simulink model "clik_z_inverse"  (R2022b)
settings: Solver=ode1  StartTime=0.0  StopTime=4  FixedStep=0.001  RelTol=1e-3
undefined symbols (not defined in the file or in its folder): DiscIntNeverNeededParam, q0, Tc
settings Model: Creator=Xp  LastModifiedBy=reube
settings SolverCC: AlgebraicLoopSolver=TrustRegion
settings DataIOCC: LimitDataPoints=on  SaveFormat=Array  SignalLoggingSaveFormat=ModelDataLogs  ReturnWorkspaceOutputs=off
settings OptimizationCC: ExpressionDepthLimit=2147483647  InitFltsAndDblsToZero=on  LifeSpan=inf
settings DebuggingCC: SaveWithParameterizedLinksMsg=none  UnderspecifiedInitializationDetection=Classic  MergeDetectMultiDrivingBlocksExec=none  SolverPrmCheckMsg=warning  MultiTaskDSMMsg=warning  MultiTaskCondExecSysMsg=none  FcnCallInpInsideContextMsg=warning  UnconnectedInputMsg=warning  UnconnectedOutputMsg=warning  UnconnectedLineMsg=warning  StateNameClashWarn=warning  SFUnexpectedBacktrackingDiag=warning  SFNoUnconditionalDefaultTransitionDiag=warning  SFExecutionAtInitializationDiag=none  SFMachineParentedDataDiag=warning  ArithmeticOperatorsInVariantConditions=warning
settings HardwareCC: ProdBitPerPointer=32  ProdBitPerSizeT=32  ProdBitPerPtrDiffT=32  ProdLargestAtomicFloat=None  ProdIntDivRoundTo=Undefined  ProdEndianess=Unspecified  ProdWordSize=32  ProdHWDeviceType=32-bit Generic
settings ModelReferenceCC: EnableRefExpFcnMdlSchedulingChecks=on  PropagateSignalLabelsOutOfModel=off
settings SFSimCC: CustomCodeUndefinedFunction=UseInterfaceOnly
settings RTWCC: DLArmComputeVersion=19.05
settings CodeAppCC: StateflowObjectComments=on
settings GRTTargetCC: TargetLangStandard=C89/C90 (ANSI)  CombineOutputUpdateFcns=off  GRTInterface=on
settings ConfigComp: CovMetricSettings=dw  CovSaveCumulativeToWorkspaceVar=on  CovSaveSingleToWorkspaceVar=on

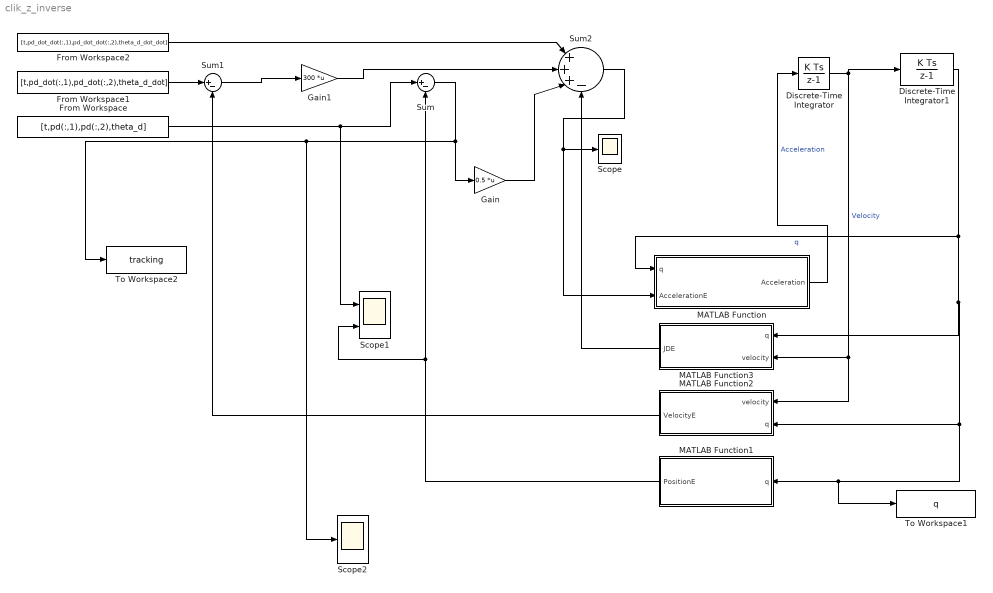
== system clik_z_inverse ==
  Discrete-Time Integrator : DiscreteIntegrator  SampleTime=Tc  ICPrevOutput=DiscIntNeverNeededParam  ICPrevScaledInput=DiscIntNeverNeededParam
  Discrete-Time Integrator1 : DiscreteIntegrator  InitialCondition=q0  SampleTime=Tc  LimitOutput=on  UpperSaturationLimit=[pi/2; pi/4; 1; 2*pi]  LowerSaturationLimit=[-pi/2; -pi/2; 0.25; -2*pi]  ICPrevOutput=DiscIntNeverNeededParam  ICPrevScaledInput=DiscIntNeverNeededParam
  From Workspace : FromWorkspace  VariableName=[t,pd(:,1),pd(:,2),theta_d]  SampleTime=Tc
  From Workspace1 : FromWorkspace  VariableName=[t,pd_dot(:,1),pd_dot(:,2),theta_d_dot]  SampleTime=Tc
  From Workspace2 : FromWorkspace  VariableName=[t,pd_dot_dot(:,1),pd_dot_dot(:,2),theta_d_dot_dot]  SampleTime=Tc
  Gain : Gain  Gain=0.5  Multiplication=Matrix(K*u)
  Gain1 : Gain  Gain=300  Multiplication=Matrix(K*u)
  MATLAB Function : MATLAB Function  TreatAsAtomicUnit=on
  MATLAB Function1 : MATLAB Function  TreatAsAtomicUnit=on
  MATLAB Function2 : MATLAB Function  TreatAsAtomicUnit=on
  MATLAB Function3 : MATLAB Function  TreatAsAtomicUnit=on
  Scope : Scope
  Scope1 : Scope  NumInputPorts=2
  Scope2 : Scope
  Sum : Sum  Inputs=|+-
  Sum1 : Sum  Inputs=|+-
  Sum2 : Sum  Inputs=|+++-
  To Workspace1 : ToWorkspace  VariableName=q  SampleTime=Tc
  To Workspace2 : ToWorkspace  VariableName=tracking  SampleTime=Tc
  wires:
  Discrete-Time Integrator1/1 -> To Workspace1/1, MATLAB Function1/1(q), MATLAB Function2/2(q), MATLAB Function3/1(q), MATLAB Function/1(q)  "q"
  MATLAB Function2/1(VelocityE) -> Sum1/2
  MATLAB Function3/1(JDE) -> Sum2/4
  Sum2/1 -> MATLAB Function/2(AccelerationE), Scope/1
  Sum1/1 -> Gain1/1
  From Workspace1/1 -> Sum1/1
  Gain/1 -> Sum2/3
  From Workspace/1 -> Sum/1, Scope1/1
  Discrete-Time Integrator/1 -> Discrete-Time Integrator1/1, MATLAB Function3/2(velocity), MATLAB Function2/1(velocity)  "Velocity"
  MATLAB Function1/1(PositionE) -> Scope1/2, Sum/2
  Gain1/1 -> Sum2/2
  MATLAB Function/1(Acceleration) -> Discrete-Time Integrator/1  "Acceleration"
  From Workspace2/1 -> Sum2/1
  Sum/1 -> Scope2/1, To Workspace2/1, Gain/1

== matlab function clik_z_inverse/MATLAB Function ==
  data: q input; Acceleration output; AccelerationE input
function Acceleration = ZRelax(q,AccelerationE)

   Jacobian = jacobian_z_relax(q);

JacobianTranspose = Jacobian';

JacobianPseusoInverse = JacobianTranspose /(Jacobian*JacobianTranspose );

I = [ 1,0,0,0;
      0,1,0,0;
      0,0,1,0
      0,0,0,1];

PseusoJacobian=(I-JacobianPseusoInverse*Jacobian);

wq =[(cos(q(2))/2)-0.2;sin(q(2)/2)+0.9;q(3)-0.3;0];

Acceleration =JacobianPseusoInverse*AccelerationE+PseusoJacobian*wq;


end

== matlab function clik_z_inverse/MATLAB Function2 ==
  data: velocity input; VelocityE output; q input
function VelocityE = Velocity(velocity,q)
    %Calculate Jacobian
%a1=0.5;
%a2 = 0.5; 
%a3 = 0;
%a4 = 0;
%alpha1 = 0;
%alpha2 = 0; 
%alpha3 = 0;
%alpha4 = 0;  
%d1 = 0;
%d2 = 0;
%d4 = 0;
%theta1 = q(1);
% theta2 = q(2);
% d3 = q(3);
% theta4 = q(4);   
        
a1 = 0.5;
a2 = 0.5;

%cos (theta1)
c1 = cos(q(1));
%sin (theta1)
s1 = sin(q(1));
%cos(theta1 + theta2)
c12 = cos(q(1)+q(2));
%sin(theta1 + theta2)
s12 = sin(q(1)+q(2));


Jacobian = [-a2*s12-a1*s1    -a2*s12   0  0; 
            a2*c12+a1*c1      a2*c12   0  0;
                  1             1      0  1];
    
   
VelocityE = transpose(Jacobian*velocity);


end

== matlab function clik_z_inverse/MATLAB Function3 ==
  data: q input; JDE output; velocity input
function JDE = Diffrential(q,velocity)
    a1 = 0.5;
    a2 = 0.5;

    
    t1 = q(1);
    t2 = q(2);
    d3 = q(3);
    t4= q(4);

    t1d = velocity(1);
    t2d = velocity(2);
    d3dot = velocity(3);
    t4d = velocity(4);




JacobianDiffrential = jacobian_dot(q,velocity);


JDE = transpose(JacobianDiffrential*velocity);


end

== matlab function clik_z_inverse/MATLAB Function1 ==
  data: q input; PositionE output
function PositionE = Kinematics(q)   
     X = direct_kin(q);

    Error = X(1:2,4);
    Error = Error';
    O = q(1) + q(2) + q(4);
    PositionE = [Error O];


    
end
